simulink model "PI_Controller"  (R2020b)
settings: Solver=VariableStepAuto  StartTime=0.0  StopTime=10  RelTol=1e-3
undefined symbols (not defined in the file): Ki, Kp
settings Model: DataDictionary=cruise.sldd  Creator=priyaD  LastModifiedBy=priyaD
settings DataIOCC: SaveOutput=off  SaveTime=off

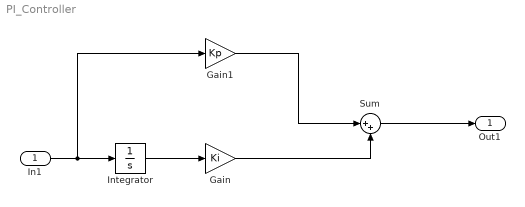
== system PI_Controller ==
  In1 : Inport  OutDataTypeStr=double  PortDimensions=1  SampleTime=0
  Gain : Gain  Gain=Ki
  Gain1 : Gain  Gain=Kp
  Integrator : Integrator
  Sum : Sum  Inputs=|++
  Out1 : Outport  OutDataTypeStr=double  PortDimensions=1  SampleTime=0
  wires:
  Gain/1 -> Sum/2
  Sum/1 -> Out1/1
  Gain1/1 -> Sum/1
  In1/1 -> Integrator/1, Gain1/1
  Integrator/1 -> Gain/1
